simulink model "MPC_with_PI"  (R2021b)
settings: Solver=VariableStepAuto  StartTime=0.0  StopTime=115  FixedStep=0.1  RelTol=1e-2
InitFcn:
  | clear all;
  | 
  | 
  | %Path in global coordinate reference frame - X and Y
  | 
  | xRef=[
  | 57.222
  | 52.707
  | 48.874
  | 44.359
  | 39.930
  | 35.160
  | 31.071
  | 16.591
  | 7.391
  | -2.575
  | -9.901
  | -13.563
  | -16.289
  | -17.567
  | -15.437
  | -8.538
  | -2.745
  | 1.002
  | 6.624
  | 10.628
  | 15.654
  | 20.935
  | 24.853
  | 28.260
  | 31.327
  | 33.797
  | 35.841
  | 36.182
  | 35.671
  | 34.478
  | 32.008
  | 29.964
  | 28.005
  | 26.301
  | 25.109
  | 24.001
  | 23.149
  | 22.383
  | 21.957
  | 21.531
  | 21.190
  | 20.850
  | 20.594
  | 21.105
  | 21.531
  | 21.701
  | 21.701
  | 21.531
  | 21.361
  | 21.446
  | 22.042
  | 23.831
  | 25.875
  | 28.771
  | ... (+154 lines)
libraries: autolibutils x4, autolibshared x2, sim3dlib x2, vehdynlibviscommon x1, slpidlib x1, simulink x1, vdynlib x1, vehdynlibsteering x1, eeGeneralControl x1, dspvision x1
(part 3 of 3)

== matlab function MPC_with_PI/MATLAB Function ==
  data: x input; Steering_Angle output; y input; yaw input; cx input; cy input; cyaw input; velocity_target input; Wheelbase input; velocity_optimal output; Steering_ratio input
function [Steering_Angle,velocity_optimal] = mpc_control(x,y,yaw,cx,cy,cyaw,velocity_target,Wheelbase,Steering_ratio) 

dt=0.01;
%figuring out the nearest point on the path
N =  length(cx);
Distance = zeros(N,1);
for i = 1:N
Distance(i) =  sqrt((cx(i)-x)^2 + (cy(i)-y)^2);
end
[~, ind]= min(Distance); %getting the index of nearest point


angle=cyaw(ind); %figuring out the target yaw angle in global reference frame
mat=[cos(angle) -sin(angle);
        sin(angle) cos(angle)]; %calculating transformation mat
p = [cx, cy]; %location vector
p= p*mat; %applying transformation - aligning with car's reference frame
pd=zeros(length(cx)-1);
pdd=zeros(length(cx)-2);
k=zeros(length(cx)-1);



for i = 1:length(cx)-1
pd(i) = (p(i+1,2)-p(i,2))/(p(i+1,1)-p(i,1));
end
%calculating the curvature
for i =2: length(cx)-1
pdd(i) = (p(i+1,2)-2*p(i,2) + p(i-1,2))/(0.5*(-p(i-1,1)+p(i+1,1)))^2;
end
for i  = 1:length(cx)-1
k(i) = (pdd(i))/(1+pd(i)^2)^(1.5);
end

vd1=velocity_target;
k =k(ind);
vd2=atan(Wheelbase * k);

    Nx=3;%number of states
    Nu =2;%number of controls
    Np =60;%prediction horizon
    Nc=30;%Control horizon
    Q=kron(eye(Np),diag([3 60 45]));   
    R=50*eye(Nc*Nu);
    kesi=zeros(Nx+Nu,1);
    kesi(1)=x-cx(ind);%error in x index
    kesi(2)=y-cy(ind);%error in y index
    kesi(3)=yaw-cyaw(ind); %error in yaw index
    kesi(4)=0.1;
    kesi(5)=0.1;

%mat initialization   
    A=[1    0  -vd1*sin(yaw)*dt      cos(yaw)*dt                 0;
       0    1  vd1*cos(yaw)*dt        sin(yaw)*dt                0;
       0    0      1             tan(vd2)*dt/Wheelbase      vd1*dt/(Wheelbase*(cos(vd2).^2))
       0    0      0                   1                         0
       0    0      0                   0                         1];
    B=[cos(yaw)*dt                   0;
       sin(yaw)*dt                   0;
       tan(vd2)*dt/Wheelbase      vd1*dt/(Wheelbase*(cos(vd2).^2))
       1                             0
       0                             1];
    C=[1 0 0 0 0;0 1 0 0 0;0 0 1 0 0;];
    
 
    PHI=zeros(Np*Nx,Nx+Nu);
    product=eye(Nx+Nu);
    for j=1:1:Np
        PHI((j-1)*Nx+1:j*Nx, :)=C*A(:,:)*product;
        product=A(:,:)*product;
    end
    
    THETA=zeros(Np*Nx,Nc*Nu);
    for k=1:1:Nc
        product=eye(Nx+Nu);
        for j=k:1:Np
            THETA((j-1)*Nx+1:j*Nx,(k-1)*Nu+1:k*Nu)=C*product*B(:,:);
            product=A(:,:)*product;
        end
    end

    H=THETA'*Q*THETA+R;
    H = 1/2*(H+H');
    f=2*(PHI*kesi)'*Q*THETA;

 A_t=zeros(Nc,Nc);
    for p=1:1:Nc
        for q=1:1:Nc
            if q<=p 
                A_t(p,q)=1;
            else 
                A_t(p,q)=0;
            end
        end 
    end 
    A_I=kron(A_t,eye(Nu));%Corresponding to the mat A processed by the constraints of the falcone paper, find the Kronecker product
    umin=[-5;-5];%The number of dimensions is the same as the number of control variables
    umax=[5;5];
    delta_umin = [ -5; -0.1];
    delta_umax = [  2 ; 0.1];
    Umin=kron(ones(Nc,1),umin);
    Umax=kron(ones(Nc,1),umax);
    A_cons=cat(1,A_I,-A_I);
    b_cons=cat(1,Umax,-Umin);
    delta_Umin=kron(ones(Nc,1),delta_umin);
    delta_Umax=kron(ones(Nc,1),delta_umax);
    lb=[delta_Umin];%(solving equation) lower bound of state quantity, including control increment and relaxation factor in control time domain
    ub=[delta_Umax];%（Solve the equation) upper bound of the state quantity, including the control increment and relaxation factor in the control time domain
    % Running Quadratic programming to optimize the MPC
    options = optimoptions('quadprog','Algorithm','active-set');
    X=zeros(Np,1);
    x_start=zeros(Nu*Nc,1);
    [X,~,~]=quadprog(H,f,A_cons,b_cons,[],[],lb,ub,x_start,options);
    % Formulating the output     
    velocity_optimal=X(1)+vd1;
    delta=X(2)+vd2;
    Steering_Angle=Steering_ratio*delta;
end

== matlab function MPC_with_PI/Path_smoothing_function ==
  data: u1 input; xRef output; u2 input; yRef output; yawRef output
function [xRef,yRef,yawRef] = fcn(u1,u2)

yaw=zeros(size(u1));
directionRef=ones(size(u1));
refPoses=[u1 u2 yaw];
refDirections=[directionRef];
numSmoothPoses=2000;
[poses,~] = smoothPathSpline(refPoses,refDirections,numSmoothPoses);

xRef=poses(:,1);
yRef=poses(:,2);
yawRef=poses(:,3);
yawRef=unwrap(wrapTo2Pi(yawRef*pi/180));

end
